simulink model "rotations_vs_coordsys"  (R2019b)
settings: Solver=VariableStepAuto  StartTime=0.0  StopTime=10.0  RelTol=1e-3
undefined symbols (not defined in the file): DiscIntNeverNeededParam
libraries: blocklib x4, simulink x1
settings Model: Creator=imanol  LastModifiedBy=imanol

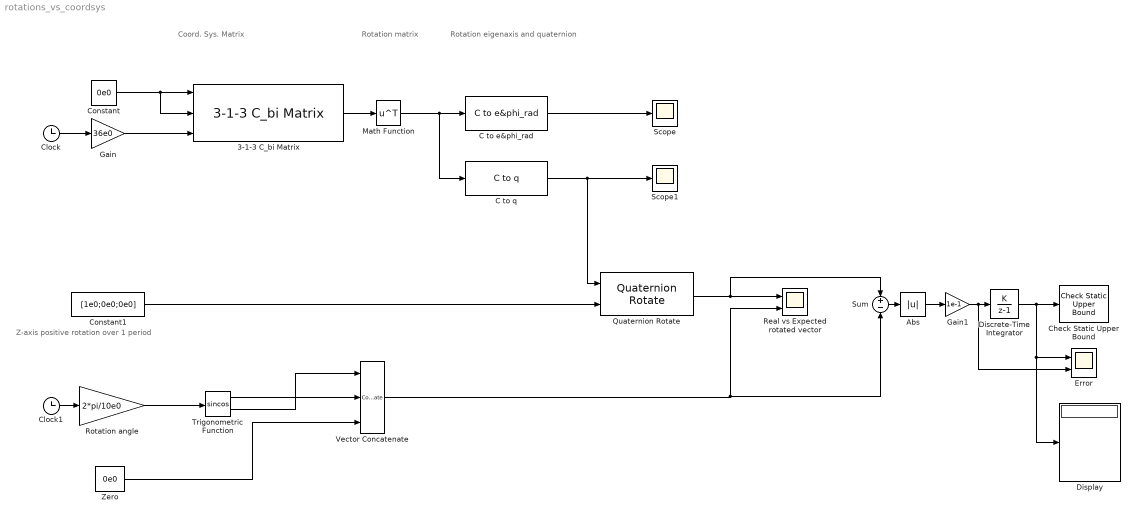
== system rotations_vs_coordsys ==
  note: Z-axis positive rotation over 1 period
  note: Rotation eigenaxis
      | and quaternion
  note: Coord. Sys. Matrix
  note: Rotation
      | matrix
  3-1-3 C_bi Matrix : blocklib/3-1-3 C_bi Matrix  Tag=|  SystemSampleTime=-1  Latency=0  AutoFrameSizeCalculation=off
      | text(.05,.5,'{\itEquation:}  \Sigma \alpha^2 + 
      | \beta^2 \rightarrow \infty, \Pi, \phi_3 = {\bfcool}', 
      | 'hor','left','texmode','on')
      settings: SourceProductName=Custom Library
  Abs : Abs  ZeroCross=off
  C to e&phi_rad : blocklib/C to e&phi_rad  SystemSampleTime=-1  Latency=0  AutoFrameSizeCalculation=off
      settings: SourceProductName=Custom Library
  C to q : blocklib/C to q  SystemSampleTime=-1  Latency=0  AutoFrameSizeCalculation=off
      settings: SourceProductName=Custom Library
  Check Static Upper Bound : simulink/Model Verification/Check Static  Upper Bound  Description=u <= 1e-6  max=1e-6  max_included=on  enabled=on  stopWhenAssertionFail=off  export=off  icon=graphic
      settings: SourceProductName=Simulink  SourceProductBaseCode=SL
  Clock : Clock
  Clock1 : Clock
  Constant : Constant  Value=0e0
  Constant1 : Constant  Value=[1e0;0e0;0e0]
  Discrete-Time Integrator : DiscreteIntegrator  IntegratorMethod=Accumulation: Forward Euler  InitialCondition=[0e0;0e0;0e0]  SampleTime=-1  ICPrevOutput=DiscIntNeverNeededParam  ICPrevScaledInput=DiscIntNeverNeededParam
  Display : Display
  Error : Scope  NumInputPorts=2
  Gain : Gain  Gain=36e0
  Gain1 : Gain  Gain=1e-1
  Math Function : Math  Operator=transpose  SignedPower=off  SaturateOnIntegerOverflow=on
  Quaternion Rotate : blocklib/Quaternion Rotate  SystemSampleTime=-1  Latency=0  AutoFrameSizeCalculation=off
      settings: SourceProductName=Custom Library
  Real vs Expected rotated vector : Scope  NumInputPorts=2
  Rotation angle : Gain  Gain=2*pi/10e0
  Scope : Scope
  Scope1 : Scope
  Sum : Sum  Inputs=+|-
  Trigonometric Function : Trigonometry  Operator=sincos
  Vector Concatenate : Concatenate  NumInputs=3
  Zero : Constant  Value=0e0
  wires:
  3-1-3 C_bi Matrix/1 -> Math Function/1
  C to e&phi_rad/1 -> Scope/1
  Clock/1 -> Gain/1
  Gain/1 -> 3-1-3 C_bi Matrix/3
  Constant/1 -> 3-1-3 C_bi Matrix/2, 3-1-3 C_bi Matrix/1
  Math Function/1 -> C to q/1, C to e&phi_rad/1
  C to q/1 -> Quaternion Rotate/1, Scope1/1
  Clock1/1 -> Rotation angle/1
  Rotation angle/1 -> Trigonometric Function/1
  Trigonometric Function/2 -> Vector Concatenate/1
  Trigonometric Function/1 -> Vector Concatenate/2
  Zero/1 -> Vector Concatenate/3
  Constant1/1 -> Quaternion Rotate/2
  Quaternion Rotate/1 -> Real vs Expected rotated vector/1, Sum/1
  Vector Concatenate/1 -> Sum/2, Real vs Expected rotated vector/2
  Sum/1 -> Abs/1
  Abs/1 -> Gain1/1
  Discrete-Time Integrator/1 -> Check Static Upper Bound/1, Error/1, Display/1
  Gain1/1 -> Error/2, Discrete-Time Integrator/1
